simulink model "SPBallonfull"  (R2024a)
settings: Solver=ode1  StartTime=0.0  StopTime=150000  FixedStep=0.1  RelTol=1e-3
settings Model: Creator=Van Chung  LastModifiedBy=Van Chung
settings SolverCC: ZeroCrossAlgorithm=Adaptive
settings DebuggingCC: IgnoredZcDiagnostic=none  UnderSpecifiedDimensionMsg=warning

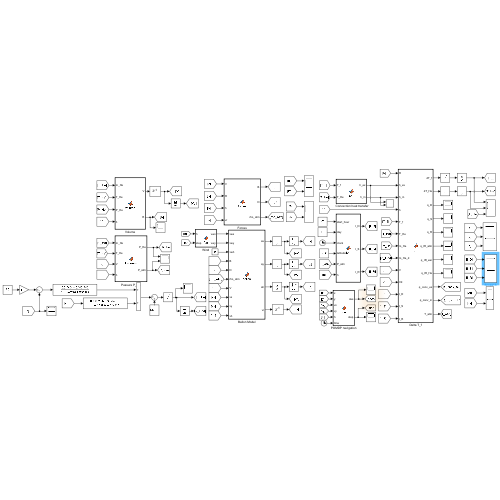
[thumbnail: Simulink's stored preview of the top-level diagram]
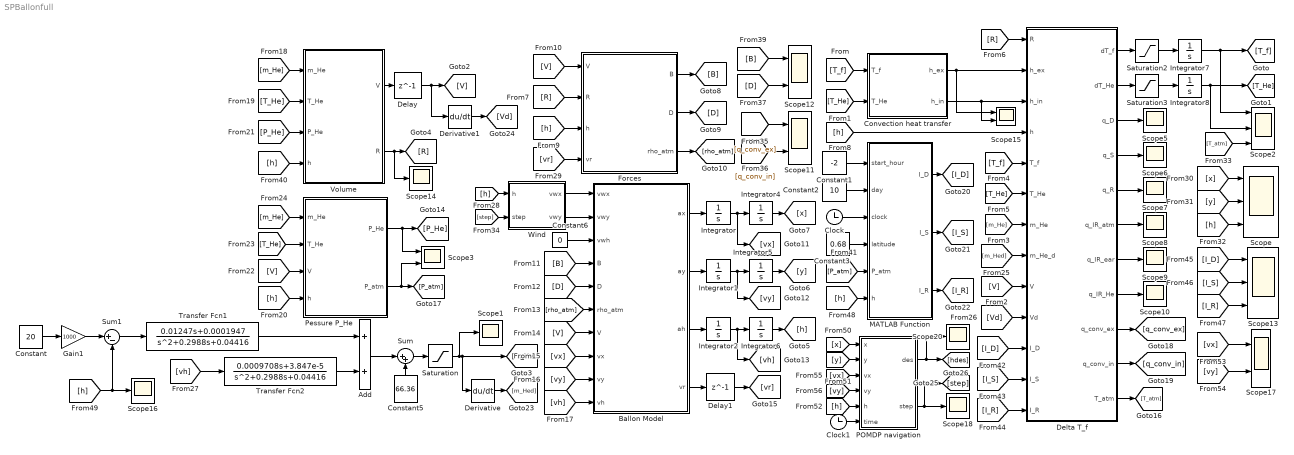
== system SPBallonfull ==
  "  Convection heat transfer" : MATLAB Function  TreatAsAtomicUnit=on
  Add : Sum
  Ballon Model : MATLAB Function  TreatAsAtomicUnit=on
  Clock : Clock
  Clock1 : Clock
  Constant : Constant  Value=20
  Constant1 : Constant  Value=-2
  Constant2 : Constant  Value=10
  Constant3 : Constant  Value=0.68
  Constant5 : Constant  Value=66.36
  Constant6 : Constant  Value=0
  Delay : Delay  DelayLength=1  InitialCondition=787.5
  Delay1 : Delay  DelayLength=1
  Delta T_f : MATLAB Function  TreatAsAtomicUnit=on
  Derivative : Derivative
  Derivative1 : Derivative
  Forces : MATLAB Function  TreatAsAtomicUnit=on
  Gain1 : Gain  Gain=1000
  Integrator : Integrator
  Integrator1 : Integrator
  Integrator2 : Integrator  UpperSaturationLimit=5  LowerSaturationLimit=-5
  Integrator4 : Integrator  LimitOutput=on  UpperSaturationLimit=20000  LowerSaturationLimit=0
  Integrator5 : Integrator  LimitOutput=on  UpperSaturationLimit=20000  LowerSaturationLimit=0
  Integrator6 : Integrator  InitialCondition=1000  LimitOutput=on  LowerSaturationLimit=0
  Integrator7 : Integrator  InitialCondition=298
  Integrator8 : Integrator  InitialCondition=298
  MATLAB Function : MATLAB Function  TreatAsAtomicUnit=on
  POMDP navigation : MATLAB Function  TreatAsAtomicUnit=on
  Pessure P_He : MATLAB Function  TreatAsAtomicUnit=on
  Saturation : Saturate  UpperLimit=85  LowerLimit=45
  Saturation2 : Saturate  UpperLimit=1  LowerLimit=-1
  Saturation3 : Saturate  UpperLimit=1  LowerLimit=-1
  Scope : Scope  NumInputPorts=3
  Scope{1,5..10,14,16,18,20} (11 alike) : Scope
  Scope{3,11..12,15,17} (5 alike) : Scope  NumInputPorts=2
  Scope13 : Scope  NumInputPorts=3
  Scope2 : Scope  NumInputPorts=3
  Sum : Sum  Inputs=|++
  Sum1 : Sum  Inputs=|+-
  Transfer Fcn1 : TransferFcn  Numerator=[0.01247 0.0001947]  Denominator=[1 0.2988 0.04416]
  Transfer Fcn2 : TransferFcn  Numerator=[0.0009708 3.847e-5]  Denominator=[1 0.2988 0.04416]
  Volume : MATLAB Function  TreatAsAtomicUnit=on
  Wind : MATLAB Function  TreatAsAtomicUnit=on
  wires:
  Ballon Model/1(ax) -> Integrator/1
  Ballon Model/3(ah) -> Integrator2/1
  Ballon Model/2(ay) -> Integrator1/1
  Volume/1(V) -> Delay/1
  Integrator/1 -> [vx], Integrator4/1
  Integrator1/1 -> [vy], Integrator5/1
  Integrator2/1 -> [vh], Integrator6/1
  Delta T_f/1(dT_f) -> Saturation2/1
  Delta T_f/2(dT_He) -> Saturation3/1
  "  Convection heat transfer"/2(h_in) -> Scope15/2, Delta T_f/3(h_in)
  "  Convection heat transfer"/1(h_ex) -> Scope15/1, Delta T_f/2(h_ex)
  [h] -> Delta T_f/4(h)
  [R] -> Delta T_f/1(R)
  [m_He] -> Delta T_f/7(m_He)
  [m_Hed] -> Delta T_f/8(m_He_d)
  [V] -> Delta T_f/9(V)
  [Vd] -> Delta T_f/10(Vd)
  Integrator7/1 -> [T_f], Scope2/1
  [T_f] -> "  Convection heat transfer"/1(T_f)
  Integrator8/1 -> [T_He], Scope2/2
  [T_He] -> "  Convection heat transfer"/2(T_He)
  [T_f] -> Delta T_f/5(T_f)
  [T_He] -> Delta T_f/6(T_He)
  Volume/2(R) -> Scope14/1, [R]
  [R] -> Forces/2(R)
  Integrator6/1 -> [h]
  Integrator5/1 -> [y]
  Integrator4/1 -> [x]
  [h] -> Forces/3(h)
  [V] -> Forces/1(V)
  Forces/1(B) -> [B]
  Forces/2(D) -> [D]
  [B] -> Ballon Model/4(B)
  [D] -> Ballon Model/5(D)
  Forces/3(rho_atm) -> [rho_atm]
  [rho_atm] -> Ballon Model/6(rho_atm)
  [V] -> Ballon Model/7(V)
  [vx] -> Ballon Model/8(vx)
  [vy] -> Ballon Model/9(vy)
  [vh] -> Ballon Model/10(vh)
  [m_He] -> Volume/1(m_He)
  [T_He] -> Volume/2(T_He)
  Pessure P_He/1(P_He) -> Scope3/1, [P_He]
  [P_He] -> Volume/3(P_He)
  [V] -> Pessure P_He/3(V)
  [T_He] -> Pessure P_He/2(T_He)
  [m_He] -> Pessure P_He/1(m_He)
  Ballon Model/4(vr) -> Delay1/1
  [vr] -> Forces/4(vr)
  Delay1/1 -> [vr]
  [x] -> Scope/1
  [y] -> Scope/2
  [h] -> Scope/3
  Delta T_f/3(q_D) -> Scope5/1
  Delta T_f/4(q_S) -> Scope6/1
  Delta T_f/5(q_R) -> Scope7/1
  Delta T_f/6(q_IR_atm) -> Scope8/1
  Delta T_f/7(q_IR_ear) -> Scope9/1
  Delta T_f/8(q_IR_He) -> Scope10/1
  Delta T_f/9(q_conv_ex) -> [q_conv_ex]
  Delta T_f/10(q_conv_in) -> [q_conv_in]
  Delta T_f/11(T_atm) -> [T_atm]
  [T_atm] -> Scope2/3
  [q_conv_ex] -> Scope11/1
  [q_conv_in] -> Scope11/2
  [D] -> Scope12/2
  [B] -> Scope12/1
  Delay/1 -> Derivative1/1, [V]
  [h] -> Pessure P_He/4(h)
  [h] -> Volume/4(h)
  Clock/1 -> MATLAB Function/3(clock)
  Constant1/1 -> MATLAB Function/1(start_hour)
  Constant2/1 -> MATLAB Function/2(day)
  Constant3/1 -> MATLAB Function/4(latitude)
  [P_atm] -> MATLAB Function/5(P_atm)
  MATLAB Function/1(I_D) -> [I_D]
  MATLAB Function/2(I_S) -> [I_S]
  MATLAB Function/3(I_R) -> [I_R]
  [I_D] -> Delta T_f/11(I_D)
  [I_S] -> Delta T_f/12(I_S)
  [I_R] -> Delta T_f/13(I_R)
  [I_R] -> Scope13/3
  [I_S] -> Scope13/2
  [I_D] -> Scope13/1
  [h] -> MATLAB Function/6(h)
  Constant/1 -> Gain1/1
  [h] -> Scope16/1, Sum1/2
  Pessure P_He/2(P_atm) -> Scope3/2, [P_atm]
  Derivative1/1 -> [Vd]
  Sum1/1 -> Transfer Fcn1/1
  Saturation/1 -> Scope1/1, Derivative/1, [m_He]
  Saturation2/1 -> Integrator7/1
  Saturation3/1 -> Integrator8/1
  Derivative/1 -> [m_Hed]
  Sum/1 -> Saturation/1
  Constant5/1 -> Sum/2
  Add/1 -> Sum/1
  Constant6/1 -> Ballon Model/3(vwh)
  Wind/1(vwx) -> Ballon Model/1(vwx)
  Wind/2(vwy) -> Ballon Model/2(vwy)
  [h] -> Wind/1(h)
  POMDP navigation/2(step) -> [step], Scope18/1
  [step] -> Wind/2(step)
  POMDP navigation/1(des) -> Scope20/1, [hdes]
  [x] -> POMDP navigation/1(x)
  [y] -> POMDP navigation/2(y)
  [h] -> POMDP navigation/5(h)
  Gain1/1 -> Sum1/1
  Clock1/1 -> POMDP navigation/6(time)
  [vx] -> Scope17/1
  [vy] -> Scope17/2
  [vx] -> POMDP navigation/3(vx)
  [vy] -> POMDP navigation/4(vy)
  Transfer Fcn2/1 -> Add/2
  Transfer Fcn1/1 -> Add/1
  [vh] -> Transfer Fcn2/1

== matlab function SPBallonfull/Delta T_f ==
  data: R input; dT_f output; h_ex input; h_in input; h input; T_f input; T_He input; dT_He output; m_He input; m_He_d input; V input; Vd input; q_D output; q_S output; q_R output; q_IR_atm output; q_IR_ear output; q_IR_He output; q_conv_ex output; q_conv_in output; T_atm output; I_D input; I_S input; I_R input
function [dT_f, dT_He, q_D, q_S, q_R, q_IR_atm, q_IR_ear, q_IR_He, q_conv_ex, q_conv_in, T_atm] = dtf(R, h_ex, h_in, h, T_f, T_He, m_He, m_He_d, V, Vd, I_D, I_S, I_R)

m_f = 181; % Mass of the film in kg
c_f = 1550; % Specific heat of the film in J/(kg*K)
alpha = 0.025; % Absorptivity of the film
A_projected = pi * R^2;
A_surf = 4 * pi * R^2; 

sigma = 5.67037442e-8; % StefanBoltzmann constant
epsilon = 0.2; %the emissivity of the polyethylene
T_ear = 288; 
tau_IR_ear = 0.95;

c_V_He = 12.75;  % in J/(mol·K)
c_P_He = 20.25;  % in J/(mol·K)

q_D = alpha * I_D * A_projected;
q_S = alpha * I_S * A_surf;
q_R = alpha * I_R * A_projected;
T_atm = calculate_atmospheric_temperature(h);

I_IR_atm = epsilon * sigma * (T_atm^4 - T_f^4);
I_IR_ear = tau_IR_ear * epsilon * sigma * (T_ear^4 - T_f^4);
I_IR_He = epsilon * sigma * (T_He^4 - T_f^4);

q_IR_atm = I_IR_atm * A_surf;
q_IR_ear = I_IR_ear * A_projected;
q_IR_He = I_IR_He * A_surf;

q_conv_ex = h_ex * A_surf * (T_atm - T_f);
q_conv_in = h_in * A_surf * (T_He - T_f);

dT_f = (q_D + q_S + q_R + q_IR_atm + q_IR_ear + q_IR_He + q_conv_ex + q_conv_in) / (m_f * c_f);
dT_He = -q_conv_in / (c_V_He * m_He) + (c_P_He / c_V_He - 1) * T_He * (m_He_d / m_He - Vd / V);

end


function T_atm = calculate_atmospheric_temperature(h)
    % Calculate atmospheric temperature based on altitude (h in meters)
    if h > 0 && h <= 11000
        % Troposphere (0 < h <= 11000 m)
        T_atm = 288 - 0.0065 * h;
    elseif h > 11000 && h <= 20000
        % Lower Stratosphere (11000 < h <= 20000 m)
        T_atm = 216.65;
    elseif h > 20000 && h <= 32000
        % Upper Stratosphere (20000 < h <= 32000 m)
        T_atm = 216.65 + 0.0010 * (h - 20000);
    else
        % Altitude out of range
        error('Altitude h must be between 0 and 32000 meters.');
    end
end

== matlab function SPBallonfull/MATLAB Function ==
  data: start_hour input; day input; I_D output; clock input; latitude input; I_S output; P_atm input; I_R output; h input
function [I_D,I_S, I_R]  = fcn(start_hour, day, clock, latitude, P_atm, h)
P_0 = 101325;
I_0 = 1367;
e_e = 0.016708;
r_e = 0.3;

start_second = start_hour * 3600;
hour = ((start_second + clock) / (24 * 3600) - round((start_second + clock) / (24*3600))) * 24 + 12;
day = mod(day + round(clock / (24*3600)), 365);
w = 0.2618 * (hour - 12);
delta = 0.4093 * (2 * pi *(284 + day) / 365);
theta_ele = asin(sin(latitude) * sin(delta) + cos(w) * cos(latitude) * cos(delta));
lambda_e = 2 * pi * (day - 1) / 365;
lambda_am = P_atm / P_0 * (sqrt(1228.6 + (613.8 * sin(w))^2 ) - 613.8 * sin(w));

tau_atm = (exp(-0.65 * lambda_am) + exp(-0.095 * lambda_am)) * (1 + 0.4 * (P_atm / P_0)^2) / 2;
tau_sc = 0.2*exp(h/10000)*sin(w);

I_D = tau_atm * I_0 * ((1 + e_e * cos(lambda_e)) / (1 - e_e ^ 2))^2;
I_S = tau_sc * I_D;
I_R = r_e * (I_D*sin(theta_ele) + I_S);

end

== matlab function SPBallonfull/Wind ==
  data: vwx output; h input; vwy output; step input
function [vwx, vwy] = fcn(h, step)
% Convert height from meters to kilometers and round
h_km = floor(h / 1000);

% Ensure h_km is within bounds [1, 5]
h_km = max(1, min(h_km, 5));

% Define wind patterns for different time periods
wind_patterns = {
        {[1, 1], [-1, 1], [1, -1], [-1, -1], [1, -1]};
        {[-1, -1], [1, -1], [-1, 1], [1, 1], [-1, -1]};
        {[-1, 1], [1, -1], [-1, -1], [1, 1], [-1, -1]};
        {[-1, 1], [1, -1], [1, 1], [-1, -1], [-1, 1]};
        {[1, 1], [1, -1], [-1, 1], [-1, -1], [-1, -1]};
        {[-1, 1], [1, 1], [1, -1], [-1, 1], [-1, -1]};
    };

% Determine time period, ensure it stays within pattern range
time_period = min(floor(step/1000) + 1, size(wind_patterns, 1));

% Retrieve wind vector based on current height and time period
wind = wind_patterns{time_period}{h_km};

% Output wind components
vwx = wind(1);
vwy = wind(2);
end

== matlab function SPBallonfull/POMDP navigation ==
  settings: updateMethod=DISCRETE
  data: des output; x input; step output; y input; vx input; vy input; h input; time input
function [des, step] = fcn(x,y, vx, vy, h, time)
    % Persistent variables declaration
    persistent epsilon epsilon_decay episode state belief prev_belief ...
               prestate actions areaSize goalState possibleWinds hdes ...
               arrival_time is_at_hdes
    
    % Initialize only once
    if isempty(epsilon)
        % Environment parameters
        areaSize = [20, 20, 5]; 
        goalState = [10, 10];  % Corrected goal position
        actions = [0, 0, 1; 0, 0, -1; 0, 0, 0];
        possibleWinds = {[-1, -1]; [-1, 1]; [1, -1]; [1, 1]};  % Unified wind directions
        
        % Exploration parameters
        epsilon = 0.975;
        epsilon_decay = 0.925;
        
        % POMDP state initialization
        episode = 0;
        state = [0, 0, 1];  % Start position within grid bounds
        belief = ones(areaSize(3), length(possibleWinds)) / length(possibleWinds);
        prev_belief = belief;
        prestate = state;
        hdes = state(3);
        arrival_time = -1;
        is_at_hdes = false;
    end

    % Convert inputs with boundary checking
    current_z = max(1, min(floor(h/1000), areaSize(3)));
    current_pos = [max(0, min(x/1000, areaSize(1))), ...
                  max(0, min(y/1000, areaSize(2))), ...
                  current_z];
    
    % Altitude status check
    if current_z == hdes
        if ~is_at_hdes
            arrival_time = time;
            is_at_hdes = true;
        end
        
        if (time - arrival_time) >= 75
            episode = episode + 1;
            state = current_pos;
            prestate = state;
            % Update wind belief based on observed velocities
            belief = updateBelief(belief, vx, vy, state(3));

            % Exploration management
            epsilon = max(epsilon * epsilon_decay, 0.001);
            
            actionIdx = chooseAction(state, belief, goalState, actions, epsilon, possibleWinds, areaSize);
            
            % Update target altitude
            hdes = state(3) + actions(actionIdx, 3);
            hdes = max(1, min(hdes, areaSize(3)));

            belief_change = max(abs(belief(:) - prev_belief(:)));
            if belief_change > 0.25
                epsilon = 0.975;  % More conservative adjustment
                fprintf('Belief update threshold crossed: %.2f\n', belief_change);
            end

            arrival_time = -1;
            is_at_hdes = false;
            prev_belief = belief;
        end
    else
        arrival_time = -1;
        is_at_hdes = false;
    end
    
    step = episode;
    des = hdes + 0.5;
end

function actionIdx = chooseAction(state, belief, goalState, actions, epsilon, possibleWinds, areaSize)
    if rand < epsilon
        actionIdx = randi(size(actions, 1));
    else
        currentZ = state(3);
        bestZ = currentZ;
        minDistance = inf;
        
        % Evaluate all altitude levels
        for z = 1:areaSize(3)
            % Get most probable wind pattern at this altitude
            [~, windIdx] = max(belief(z, :));
            predictedWind = possibleWinds{windIdx};
            
            % Predict next position with boundary constraints
            predictedXY = state(1:2) + predictedWind;
            predictedXY = max(predictedXY, [0 0]);
            predictedXY = min(predictedXY, [areaSize(1) areaSize(2)]);
            
            % Calculate distance to goal
            dist = norm(predictedXY - goalState);
            
            % Select best altitude considering both distance and altitude proximity
            if dist < minDistance || (dist == minDistance && abs(z - currentZ) < abs(bestZ - currentZ))
                minDistance = dist;
                bestZ = z;
            end
        end
        
        % Determine optimal vertical movement
        if bestZ > currentZ
            actionIdx = 1; % Ascend
        elseif bestZ < currentZ
            actionIdx = 2; % Descend
        else
            actionIdx = 3; % Maintain
        end
    end
end

function beliefNew = updateBelief(belief, vx, vy, z_level)
    possibleWinds = {[-1, -1]; [-1, 1]; [1, -1]; [1, 1]};
    alpha = 0.5;  % More stable learning rate
    
    % Calculate effective wind direction
    wind_sign = [0, 0];
    if abs(vx) >= 0.5
        wind_sign(1) = sign(vx);
    end
    if abs(vy) >= 0.5
        wind_sign(2) = sign(vy);
    end
    
    beliefNew = belief;
    match_found = false;
    
    % Exact pattern matching
    for i = 1:length(possibleWinds)
        if isequal(wind_sign, possibleWinds{i})
            beliefNew(z_level, i) = (1-alpha)*belief(z_level, i) + alpha;
            match_found = true;
        else
            beliefNew(z_level, i) = (1-alpha)*belief(z_level, i);
        end
    end
    
    % Handle partial matches with cosine similarity
    if ~match_found
        similarities = cellfun(@(w) dot(w, wind_sign)/(norm(w)*norm(wind_sign)), possibleWinds);
        [~, best_match] = max(similarities);
        beliefNew(z_level, best_match) = (1-alpha)*belief(z_level, best_match) + alpha;
    end
    
    % Normalize beliefs
    row_sum = sum(beliefNew(z_level, :));
    if row_sum > 0
        beliefNew(z_level, :) = beliefNew(z_level, :) / row_sum;
    else
        beliefNew(z_level, :) = ones(1, length(possibleWinds))/length(possibleWinds);
    end
end

== matlab function SPBallonfull/Ballon Model ==
  data: ax output; ay output; ah output; vwx input; vwy input; vwh input; B input; D input; rho_atm input; V input; vx input; vy input; vh input; vr output
function [ax, ay, ah, vr] = ballon(vwx, vwy, vwh, B, D, rho_atm, V, vx, vy, vh)
m = 484;
g = 9.80;
Cv = 0.5;
vrx = vwx - vx;
vry = vwy - vy;
vrh = vwh - vh;
vr = (vrx^2 + vry^2 + vrh^2)^0.5;
Dx = D * vrx / vr;
Dy = D * vry / vr;
Dh = D * vrh / vr;
madd = Cv * rho_atm * V;
ax = Dx / (m + madd);
ay = Dy / (m + madd);
ah = (Dh + B - m*g) / (m + madd);
end

== matlab function SPBallonfull/  Convection heat transfer ==
  data: T_f input; h_ex output; h_in output; T_He input
function [h_ex,h_in] = chf(T_f , T_He)
Nu = 8; % Natural convection Nusselt number
k_atm = 0.026; % Thermal conductivity of atmosphere in W/(m*K)
L_0 = 12; % Characteristic length of balloon in m
Re = 288000; % Reynolds number of stratospheric balloon
k_He = 0.0015; % Thermal conductivity of Helium in W/(m*K)
rho_He = 0.1786; % Density of Helium in kg/m^3
Pr_He = 0.67; % Prandtl number of Helium
mu_He = 1.1e-4; % kinetic viscosity of helium
g = 9.80; % Gravitational acceleration in m/s^2

h_natural_ex = (Nu * k_atm) / L_0;  
% Calculate forced convective heat transfer coefficient
h_forced_ex = (2 + 0.41 * Re^0.55) * k_atm / L_0;
    
% Calculate external convective heat transfer coefficient
h_ex = (h_natural_ex^3 + h_forced_ex^3)^(1/3);
    
% Calculate internal convective heat transfer coefficient
h_in = 0.13 * k_He * ((rho_He^2 * g * abs(T_f - T_He) * Pr_He) / (T_He * mu_He^2))^(1/3);
end

== matlab function SPBallonfull/Pessure P_He ==
  data: m_He input; T_He input; P_He output; V input; h input; P_atm output
function [P_He, P_atm] = Pessure(m_He, T_He, V, h)

    R_He = 2077.1; % Specific gas constant for Helium in J/(kg*K)

    P_atm = calculate_atmospheric_pressure(h);
    % Validate inputs to prevent division by zero
    if V <= 0
        error('Volume must be greater than zero.');
    end

    if V >= 7237
        P_He = (m_He * R_He * T_He) / V;
    else
        P_He = P_atm;
    end
end

function P_atm = calculate_atmospheric_pressure(h)
    % Calculate atmospheric pressure based on altitude (h in meters)
    if h > 0 && h <= 11000
        % Troposphere (0 < h <= 11000 m)
        P_atm = 101325 * ((288 - 0.0065 * h) / 288)^5.25;
    elseif h > 11000 && h <= 20000
        % Lower Stratosphere (11000 < h <= 20000 m)
        P_atm = 22632 * exp(-(h - 11000) / 6341.62);
    elseif h > 20000 && h <= 32000
        % Upper Stratosphere (20000 < h <= 32000 m)
        P_atm = 5474.87 * ((216.65 + 0.0010 * (h - 20000)) / 216.65)^-34.163;
    else
        % Altitude out of range
        error('Altitude h must be between 0 and 32000 meters.');
    end
end

== matlab function SPBallonfull/Volume ==
  data: m_He input; V output; T_He input; P_He input; R output; h input
function [V,R] = volume(m_He, T_He, P_He, h)
    R_He = 2077; % Specific gas constant for Helium in J/(kg*K)
    
    V = (m_He * R_He * T_He) / P_He; % Volume when deltaP = 0

    d = 0.1 / 1000; % Thickness of the film in meters (0.1 mm converted to meters)
    E = 0.2e13; % Elastic modulus of the film in Pascals (0.2 GPa)
    R_0 = 12;
    P_atm = calculate_atmospheric_pressure(h);
    
    % Calculate pressure difference (deltaP)
    deltaP = P_He - P_atm;
    
    % Calculate stress (sigma_f) and strain (epsilon_f)
    if deltaP == 0
        sigma_f = 0;
    else
        sigma_f = (deltaP * R_0) / (2 * d); 
    end
    epsilon_f = sigma_f / E; % Strain in the film
    
    % Calculate actual radius (R)
    R = (1 + epsilon_f) * R_0;

    if V >= 7153
        V = 4/3 * pi * R^3;
    end
end


function P_atm = calculate_atmospheric_pressure(h)
    % Calculate atmospheric pressure based on altitude (h in meters)
    if h > 0 && h <= 11000
        % Troposphere (0 < h <= 11000 m)
        P_atm = 101325 * ((288 - 0.0065 * h) / 288)^5.25;
    elseif h > 11000 && h <= 20000
        % Lower Stratosphere (11000 < h <= 20000 m)
        P_atm = 22632 * exp(-(h - 11000) / 6341.62);
    elseif h > 20000 && h <= 32000
        % Upper Stratosphere (20000 < h <= 32000 m)
        P_atm = 5474.87 * ((216.65 + 0.0010 * (h - 20000)) / 216.65)^-34.163;
    else
        % Altitude out of range
        error('Altitude h must be between 0 and 32000 meters.');
    end
end

== matlab function SPBallonfull/Forces ==
  data: V input; B output; R input; h input; D output; vr input; rho_atm output
function [B, D, rho_atm] = forces(V,R,h, vr)
g = 9.8;
Cd = 0.8;
S = 2 * pi * R^2; 
P_atm = calculate_atmospheric_pressure(h);
T_atm = calculate_atmospheric_temperature(h);
R_m_atm = 287;
rho_atm = P_atm / (R_m_atm * T_atm);
B = rho_atm * g * V;
D = 0.5 * rho_atm * vr ^ 2 * Cd * S;
end

function T_atm = calculate_atmospheric_temperature(h)
    % Calculate atmospheric temperature based on altitude (h in meters)
    if h > 0 && h <= 11000
        % Troposphere (0 < h <= 11000 m)
        T_atm = 288 - 0.0065 * h;
    elseif h > 11000 && h <= 20000
        % Lower Stratosphere (11000 < h <= 20000 m)
        T_atm = 216.65;
    elseif h > 20000 && h <= 32000
        % Upper Stratosphere (20000 < h <= 32000 m)
        T_atm = 216.65 + 0.0010 * (h - 20000);
    else
        % Altitude out of range
        error('Altitude h must be between 0 and 32000 meters.');
    end
end


function P_atm = calculate_atmospheric_pressure(h)
    % Calculate atmospheric pressure based on altitude (h in meters)
    if h > 0 && h <= 11000
        % Troposphere (0 < h <= 11000 m)
        P_atm = 101325 * ((288 - 0.0065 * h) / 288)^5.25;
    elseif h > 11000 && h <= 20000
        % Lower Stratosphere (11000 < h <= 20000 m)
        P_atm = 22632 * exp(-(h - 11000) / 6341.62);
    elseif h > 20000 && h <= 32000
        % Upper Stratosphere (20000 < h <= 32000 m)
        P_atm = 5474.87 * ((216.65 + 0.0010 * (h - 20000)) / 216.65)^-34.163;
    else
        % Altitude out of range
        error('Altitude h must be between 0 and 32000 meters.');
    end
end
